simulink model "solartracker"  (R2022b)
settings: Solver=VariableStepAuto  StartTime=0.0  StopTime=86400  FixedStep=0.1  MaxStep=1  RelTol=1e-5
InitFcn:
  | clear all
  | clc
  | %% PARAMETERS OF DC MOTOR
  | R=18.2214;
  | L=0.000866;
  | Kb=0.030941093;
  | Km=0.030941093;
  | J=0.00009;
  | B1=0.000025;
  | 
  | %% LOADING MPC
  | load mpc1.mat
undefined symbols (not defined in the file or in its folder): DiscIntNeverNeededParam
libraries: mpclib x2
settings Model: SimulationMode=accelerator  Creator=faraj  LastModifiedBy=Sadaf
settings SolverCC: ExtrapolationOrder=1  MaxConsecutiveMinStep=50
settings DataIOCC: SaveOutput=off  SignalLogging=off  DSMLogging=off  SaveTime=off  ReturnWorkspaceOutputs=off
settings ModelReferenceCC: EnableRefExpFcnMdlSchedulingChecks=on  PropagateSignalLabelsOutOfModel=off
settings GRTTargetCC: TargetLangStandard=C89/C90 (ANSI)

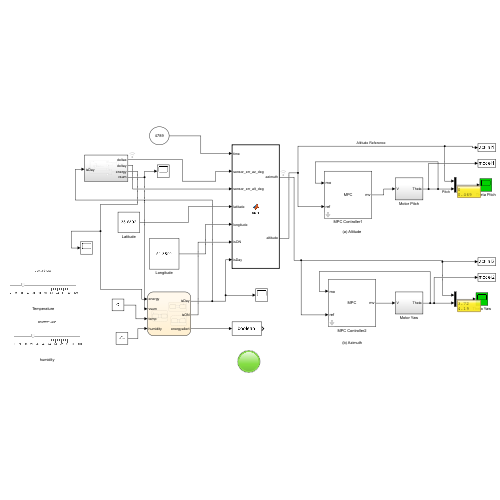
[thumbnail: Simulink's stored preview of the top-level diagram]
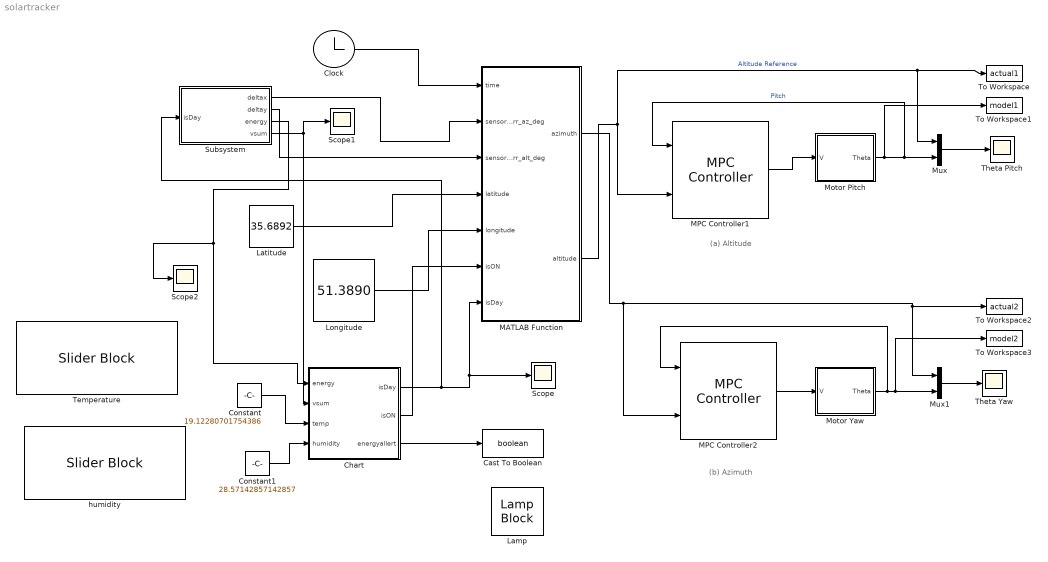
== system solartracker ==
  note: (a) Altitude
  note: (b) Azimuth
  Cast To Boolean : DataTypeConversion  OutDataTypeStr=boolean  SaturateOnIntegerOverflow=off  RndMeth=Floor
  Chart : Stateflow chart  TreatAsAtomicUnit=on
      settings: PortSchema="{\"entries\":[{\"content\":{\"sides\":[{\"content\":{\"connectorIds\":[\"In2\",\"In1\",\"In3\",\"In4\"]},\"type\":\"ConnectorPlacement.EquallySpacedRectSide\",\"uuid\":\"41b4ae27-8045-4c31-a79d-117f38c1fd05\"},{\"content\":{\"connectorIds\":[\"Out1\",\"Out2\",\"Out3\"],\"side\":\"RIGHT\"},\"type\":\"ConnectorPlacement.EquallySpacedRectSide\",\"uuid\":\"bf5803f2-d673-4cdf-83cf-d38121fbf371\"},{\"content\":{\"connectorIds\":[],\"side\":\"TOP\"},\"type\":\"ConnectorPlacement.EquallySpacedRectSide\",\"uuid\":\"83405226-3af2-4fbf-b1d9-fd19ac5e36f2\"}]},\"type\":\"ConnectorPlacement.EquallySpacedConnector\",\"uuid\":\"f3113742-9519-481f-9b9f-49de96e707b4\"}],\"packageUris\":[\"http://schema.mathworks.com/mf0/Connector/R2020b\"],\"version\":\"1.0\"}"
  Clock : Clock
      settings: Decimation=86400*121
  Constant : Constant  Value=19.12280701754386
  Constant1 : Constant  Value=28.57142857142857
  Lamp : LampBlock  LabelPosition=Hide
  Latitude : Constant  Value=35.6892
  Longitude : Constant  Value=51.3890
  MATLAB Function : MATLAB Function  TreatAsAtomicUnit=on
  MPC Controller1 : mpclib/MPC Controller  SCDEnableBlockLinearizationSpecification=on  mpcobj=mpc1  is_multiple=0  enable_value=0  return_u0=off  updateMPCinCallerWorkspace=on  md_inport=off  mv_inport=off  uref_inport=off  return_cost=off  return_mvseq=off  return_qpstatus=off  return_xseq=off  return_state=off  return_ovseq=off  state_inport=off  umin_inport=off  umax_inport=off  ymin_inport=off  ymax_inport=off  cc_inport=off  ywt_inport=off  uwt_inport=off  duwt_inport=off  rhoeps_inport=off  pm_inport=off  MaximumP=10  HorizonChoice=FixedHorizon  n_ts=0.1  n_p=10  n_mv=1  n_md=0  n_ud=0  n_mo=1  n_uo=0  BlockDataType=double  SampleTimeInherited=off  switch_inport=off
  MPC Controller2 : mpclib/MPC Controller  SCDEnableBlockLinearizationSpecification=on  mpcobj=mpc1  is_multiple=0  enable_value=0  return_u0=off  updateMPCinCallerWorkspace=on  md_inport=off  mv_inport=off  uref_inport=off  return_cost=off  return_mvseq=off  return_qpstatus=off  return_xseq=off  return_state=off  return_ovseq=off  state_inport=off  umin_inport=off  umax_inport=off  ymin_inport=off  ymax_inport=off  cc_inport=off  ywt_inport=off  uwt_inport=off  duwt_inport=off  rhoeps_inport=off  pm_inport=off  MaximumP=10  HorizonChoice=FixedHorizon  n_ts=0.1  n_p=10  n_mv=1  n_md=0  n_ud=0  n_mo=1  n_uo=0  BlockDataType=double  SampleTimeInherited=off  switch_inport=off
  Motor Pitch : Subsystem
  Motor Yaw : Subsystem
  Mux : Mux  Inputs=2
  Mux1 : Mux  Inputs=2
  Scope : Scope
  Scope1 : Scope
  Scope2 : Scope
  Subsystem : Subsystem
  Temperature : SliderBlock
  Theta Pitch : Scope
  Theta Yaw : Scope
  To Workspace : ToWorkspace  VariableName=actual1  SampleTime=1
  To Workspace1 : ToWorkspace  VariableName=model1  SampleTime=1
  To Workspace2 : ToWorkspace  VariableName=actual2  SampleTime=1
  To Workspace3 : ToWorkspace  VariableName=model2  SampleTime=1
  humidity : SliderBlock
  wires:
  MATLAB Function/2(altitude) -> MPC Controller1/2, Mux/1, To Workspace/1  "Altitude Reference"
  Motor Pitch/1(Theta) -> MPC Controller1/1, Mux/2, To Workspace1/1  "Pitch"
  MPC Controller2/1 -> Motor Yaw/1(V)
  Mux/1 -> Theta Pitch/1
  Mux1/1 -> Theta Yaw/1
  Motor Yaw/1(Theta) -> MPC Controller2/1, To Workspace3/1, Mux1/2
  MATLAB Function/1(azimuth) -> MPC Controller2/2, To Workspace2/1, Mux1/1
  Subsystem/1(deltax) -> MATLAB Function/2(sensor_err_az_deg)
  MPC Controller1/1 -> Motor Pitch/1(V)
  Latitude/1 -> MATLAB Function/4(latitude)
  Longitude/1 -> MATLAB Function/5(longitude)
  Clock/1 -> MATLAB Function/1(time)
  Subsystem/2(deltay) -> MATLAB Function/3(sensor_err_alt_deg)
  Chart/2(isON) -> MATLAB Function/6(isON)
  Constant/1 -> Chart/3(temp)
  Constant1/1 -> Chart/4(humidity)
  Chart/3(energyallert) -> Cast To Boolean/1
  Subsystem/4(vsum) -> Scope1/1, Chart/1(vsum)
  Chart/1(isDay) -> Subsystem/1(isDay), Scope/1, MATLAB Function/7(isDay)
  Subsystem/3(energy) -> Scope2/1, Chart/2(energy)

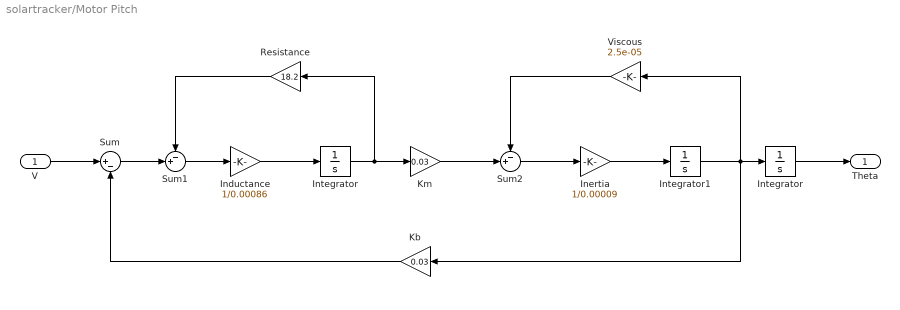
== system solartracker/Motor Pitch ==
  V : Inport
  Inductance : Gain  Gain=1/0.00086
  Inertia : Gain  Gain=1/0.00009
  Integrator : Integrator
  "Integrator " : Integrator
  Integrator1 : Integrator
  Kb : Gain  Gain=0.03
  Km : Gain  Gain=0.03
  Resistance : Gain  Gain=18.2
  Sum : Sum  Inputs=|+-
  Sum1 : Sum  Inputs=-+|
  Sum2 : Sum  Inputs=-+|
  Viscous : Gain  Gain=2.5e-05
  Theta : Outport
  wires:
  Km/1 -> Sum2/2
  Kb/1 -> Sum/2
  Inductance/1 -> Integrator/1
  Sum2/1 -> Inertia/1
  Integrator/1 -> Resistance/1, Km/1
  Integrator1/1 -> Kb/1, Viscous/1, "Integrator "/1
  Sum/1 -> Sum1/2
  Sum1/1 -> Inductance/1
  Viscous/1 -> Sum2/1
  Inertia/1 -> Integrator1/1
  Resistance/1 -> Sum1/1
  V/1 -> Sum/1
  "Integrator "/1 -> Theta/1

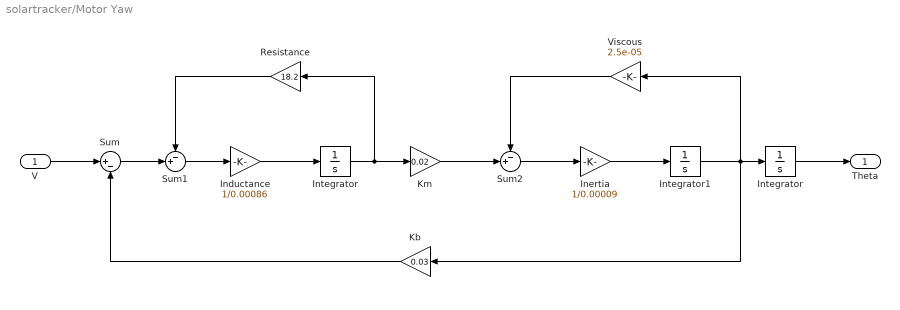
== system solartracker/Motor Yaw ==
  V : Inport
  Inductance : Gain  Gain=1/0.00086
  Inertia : Gain  Gain=1/0.00009
  Integrator : Integrator
  "Integrator " : Integrator
  Integrator1 : Integrator
  Kb : Gain  Gain=0.03
  Km : Gain  Gain=0.02
  Resistance : Gain  Gain=18.2
  Sum : Sum  Inputs=|+-
  Sum1 : Sum  Inputs=-+|
  Sum2 : Sum  Inputs=-+|
  Viscous : Gain  Gain=2.5e-05
  Theta : Outport
  wires:
  Km/1 -> Sum2/2
  Kb/1 -> Sum/2
  Inductance/1 -> Integrator/1
  Sum2/1 -> Inertia/1
  Integrator/1 -> Resistance/1, Km/1
  Integrator1/1 -> Kb/1, Viscous/1, "Integrator "/1
  Sum/1 -> Sum1/2
  Sum1/1 -> Inductance/1
  Viscous/1 -> Sum2/1
  Inertia/1 -> Integrator1/1
  Resistance/1 -> Sum1/1
  V/1 -> Sum/1
  "Integrator "/1 -> Theta/1

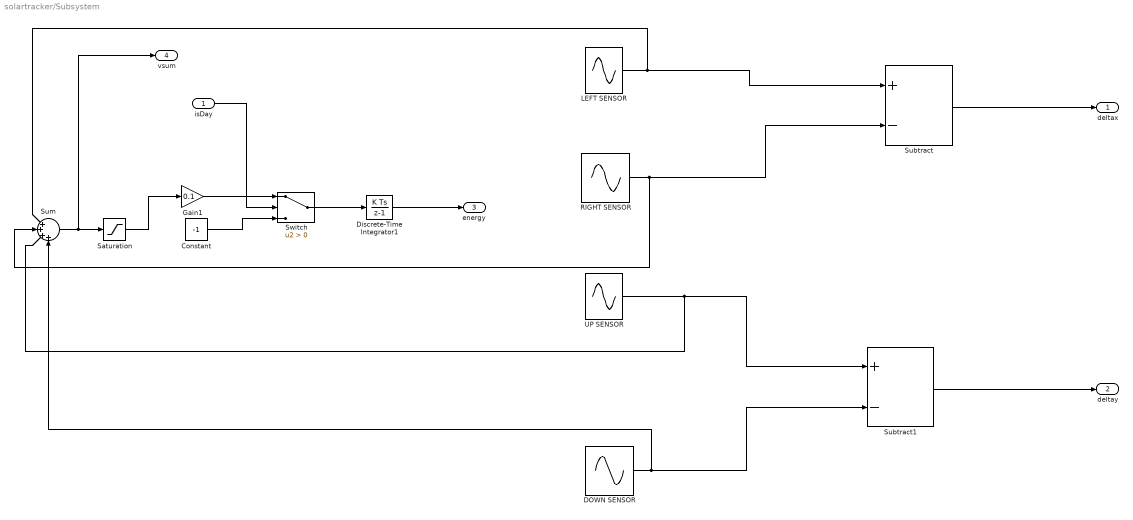
== system solartracker/Subsystem ==
  isDay : Inport
  Constant : Constant  Value=-1
  DOWN SENSOR : Sin  Amplitude=0.5  Bias=0.5  Frequency=0.00004  SampleTime=0
  Discrete-Time Integrator1 : DiscreteIntegrator  gainval=1/3600  SampleTime=-1  LimitOutput=on  UpperSaturationLimit=1  LowerSaturationLimit=0  ICPrevOutput=DiscIntNeverNeededParam  ICPrevScaledInput=DiscIntNeverNeededParam
  Gain1 : Gain  Gain=0.1
  LEFT SENSOR : Sin  Amplitude=0.5  Bias=0.5  Frequency=0.00004  SampleTime=0
  RIGHT SENSOR : Sin  Amplitude=0.5  Bias=0.5  Frequency=0.00004  SampleTime=0
  Saturation : Saturate  UpperLimit=1  LowerLimit=0
  Subtract : Sum  Inputs=+-
  Subtract1 : Sum  Inputs=+-
  Sum : Sum  Inputs=|++++
  Switch : Switch  Criteria=u2 > Threshold  SaturateOnIntegerOverflow=off  InputSameDT=off
  UP SENSOR : Sin  Amplitude=0.5  Bias=0.5  Frequency=0.00004  SampleTime=0
  deltax : Outport
  deltay : Outport  Port=2
  energy : Outport  Port=3
  vsum : Outport  Port=4
  wires:
  LEFT SENSOR/1 -> Sum/1, Subtract/1
  RIGHT SENSOR/1 -> Subtract/2, Sum/2
  DOWN SENSOR/1 -> Subtract1/2, Sum/4
  UP SENSOR/1 -> Sum/3, Subtract1/1
  Subtract/1 -> deltax/1
  Subtract1/1 -> deltay/1
  Sum/1 -> vsum/1, Saturation/1
  Saturation/1 -> Gain1/1
  Gain1/1 -> Switch/1
  Switch/1 -> Discrete-Time Integrator1/1
  Constant/1 -> Switch/3
  Discrete-Time Integrator1/1 -> energy/1
  isDay/1 -> Switch/2

== matlab function solartracker/MATLAB Function ==
  settings: updateMethod=DISCRETE
  data: time input; azimuth output; altitude output; sensor_err_az_deg input; sensor_err_alt_deg input; latitude input; longitude input; isON input; isDay input
function [azimuth, altitude] = sun(time, sensor_err_az_deg, sensor_err_alt_deg, latitude, longitude, isON, isDay)
% Outputs are in radians (azimuth in [0,2π), altitude in [0, π/2]).
% time: seconds (real time). latitude/longitude: degrees.

    persistent lastAz lastAlt
    if isempty(lastAz),  lastAz  = 0.0; end
    if isempty(lastAlt), lastAlt = 0.0; end

    azimuth  = lastAz;
    altitude = lastAlt;

    if isON && isDay
        dayLength = 86400;                                    % 24*60*60
        nt = mod(time, dayLength) / dayLength;                % [0..1)

   
        declination = 23.45 * sind( 360 * (284 + nt*365.25) / 365 );  % deg
        H = (nt - 0.5) * 360 + longitude;                              % hour angle (deg)
        phi = latitude;                                                % deg

        num  = sind(H);
        den  = cosd(H)*sind(phi) - tand(declination)*cosd(phi);
        az_deg = atan2d(num, den);
        if az_deg < 0, az_deg = az_deg + 360; end                      % wrap to [0,360)

        az_deg = az_deg + sensor_err_az_deg;
        if az_deg >= 360
            az_deg = az_deg - 360;
        elseif az_deg < 0
            az_deg = az_deg + 360;
        end


        el_deg = asind( sind(phi)*sind(declination) + ...
                        cosd(phi)*cosd(declination)*cosd(H) );       

        el_deg = el_deg + sensor_err_alt_deg;                  


        if     el_deg <   0, el_deg = 0;
        elseif el_deg >  90, el_deg = 90;
        end
        
        azimuth  = deg2rad(az_deg);
        altitude = deg2rad(el_deg);

        lastAz   = azimuth;
        lastAlt  = altitude;
    end
end

== stateflow chart solartracker/Chart ==
  state DayNight [parallel]
    settings: executionOrder=3
    state Day
    state Night
    (default) -> Night
    Day -> Night : [vsum/4 < 0.54]{isDay = false}
    Night -> Day : [vsum/4 > 0.56]{isDay = true}
  state EnvMonitor [parallel]
    settings: executionOrder=1
    state Functioning
    state fault
    (default) -> Functioning
    Functioning -> fault : [(temp > 50) || (humidity >80)]{isON = false}
    fault -> Functioning : [(temp < 50) && (humidity <78)]{isON = true}
  state EnergyGuard [parallel]
    settings: executionOrder=2
    state low
    state Normal
    (default) -> Normal
    Normal -> low : [energy<0.19]{energyallert = true}
    low -> Normal : [energy > 0.21]{energyallert = false}
  data: vsum input double; energy input double; temp input double; humidity input double; isDay output boolean =false; isON output boolean =true; energyallert output boolean =false
